simulink model "test_plotblock"  (R2015a)
settings: Solver=ode45  StartTime=0.0  StopTime=inf  RelTol=1e-3
undefined symbols (not defined in the file): field_x, field_y, items
libraries: visionsinks x1
settings Model: Creator=tzwijger  LastModifiedBy=tzwijger

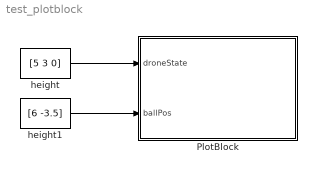
== system test_plotblock ==
  PlotBlock : Subsystem
  height : Constant  Value=[5 3 0]  SampleTime=1/20
  height1 : Constant  Value=[6 -3.5]  SampleTime=1/20
  wires:
  height/1 -> PlotBlock/1(droneState)
  height1/1 -> PlotBlock/2(ballPos)

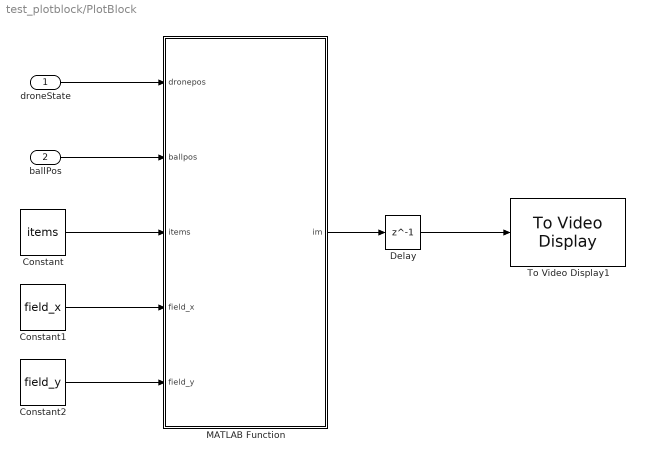
== system test_plotblock/PlotBlock ==
  droneState : Inport
  ballPos : Inport  Port=2
  Constant : Constant  Value=items
  Constant1 : Constant  Value=field_x
  Constant2 : Constant  Value=field_y
  Delay : Delay  DelayLength=1  SampleTime=1/400
  MATLAB Function : MATLAB Function  TreatAsAtomicUnit=on
  To Video Display1 : visionsinks/To Video Display  windowSizeMode=True size (1:1)  openAtMdlStart=off  fullScreen=off  videoWindowX=81  videoWindowY=111  saveWindowSize=off  videoWindowWidth=810  videoWindowHeight=542  inputColorFormat=RGB  inputType=Obsolete  imagePorts=One multidimensional signal  OutputDevice=On-screen video monitor  dataOrg=Column-major  isWindowOpen=off
  wires:
  Constant/1 -> MATLAB Function/3(items)
  ballPos/1 -> MATLAB Function/2(ballpos)
  droneState/1 -> MATLAB Function/1(dronepos)
  Constant1/1 -> MATLAB Function/4(field_x)
  Constant2/1 -> MATLAB Function/5(field_y)
  MATLAB Function/1(im) -> Delay/1
  Delay/1 -> To Video Display1/1

== matlab function test_plotblock/PlotBlock/MATLAB Function ==
  data: dronepos input; im output; ballpos input; items input; field_x input; field_y input
function im  = update_plot_trilat(dronepos, ballpos, items,field_x,field_y)
    
    persistent im_init field2im_params
    
    coder.extrinsic('init_plot_trilat_img','update_plot_trilat_img')    
        
    if (isempty(im_init)||isempty(field2im_params))
        [im_init,field2im_params] = init_plot_trilat_img(items,field_x,field_y);        
    end
    
    im = uint8(zeros(542,810,3));
    im = update_plot_trilat_img(im_init,field2im_params,ballpos,dronepos);   
end
